simulink model "propeller"  (R2021a)
settings: Solver=VariableStepAuto  StartTime=0.0  StopTime=0.05  FixedStep=0.01  RelTol=1e-3
InitFcn:
  | prop_init_set
values from neighbouring files (symbols this model uses):
  Cp_total = [Cp_1000rpm; Cp_2000rpm; Cp_3000rpm; Cp_4000rpm; Cp_5000rpm]    [prop_init_set.m]
  Ct_total = [Ct_1000rpm; Ct_2000rpm; Ct_3000rpm; Ct_4000rpm; Ct_5000rpm]    [prop_init_set.m]
settings Model: SimulationMode=accelerator  Creator=76568  LastModifiedBy=76568

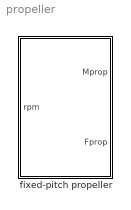
== system propeller ==
  fixed-pitch propeller : Subsystem  mask{air_speed=10, prop_diameter=0.473, T_static=16.1936, T_max=6.85, V_max=15, air_rho=1.225}

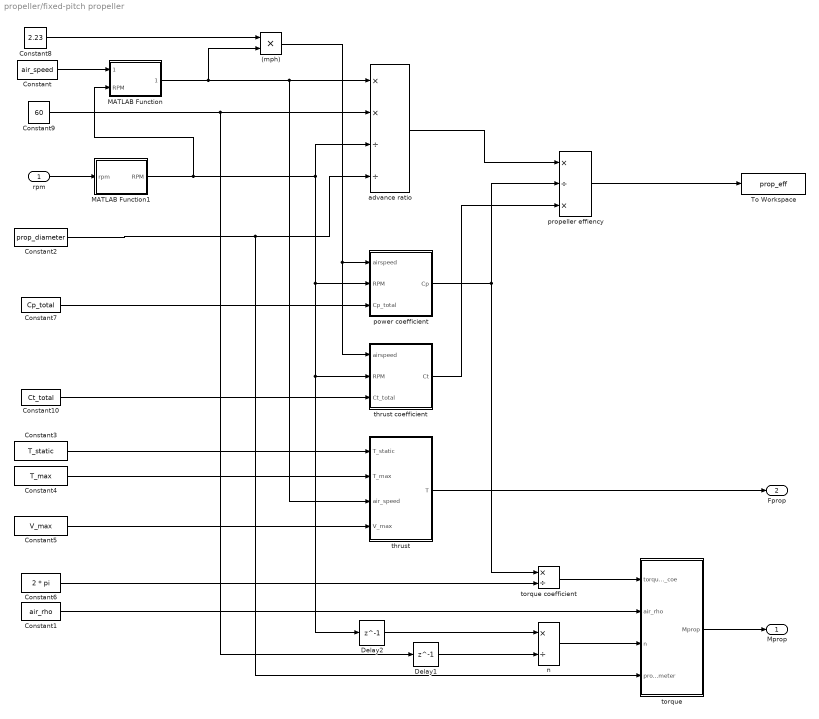
== system propeller/fixed-pitch propeller ==
  rpm : Inport
  (mph) : Product
  Constant : Constant  Value=air_speed
  Constant1 : Constant  Value=air_rho
  Constant10 : Constant  Value=Ct_total
  Constant2 : Constant  Value=prop_diameter
  Constant3 : Constant  Value=T_static
  Constant4 : Constant  Value=T_max
  Constant5 : Constant  Value=V_max
  Constant6 : Constant  Value=2 * pi
  Constant7 : Constant  Value=Cp_total
  Constant8 : Constant  Value=2.23
  Constant9 : Constant  Value=60
  Delay1 : Delay  DelayLength=1  InitialCondition=0  SampleTime=0.0001
  Delay2 : Delay  DelayLength=1  InitialCondition=0  SampleTime=0.0001
  MATLAB Function : MATLAB Function  TreatAsAtomicUnit=on
  MATLAB Function1 : MATLAB Function  TreatAsAtomicUnit=on
  To Workspace : ToWorkspace  VariableName=prop_eff  SaveFormat=Timeseries  SampleTime=-1
  advance ratio : Product  Inputs=**//
  n : Product  Inputs=*/
  power coefficient : MATLAB Function  TreatAsAtomicUnit=on
  propeller effiency : Product  Inputs=*/*
  thrust : MATLAB Function  TreatAsAtomicUnit=on
  thrust coefficient : MATLAB Function  TreatAsAtomicUnit=on
  torque : MATLAB Function  TreatAsAtomicUnit=on
  torque coefficient : Product  Inputs=*/
  Mprop : Outport
  Fprop : Outport  Port=2
  wires:
  thrust coefficient/1(Ct) -> propeller effiency/3
  MATLAB Function1/1(RPM) -> MATLAB Function/2(RPM), Delay2/1, thrust coefficient/2(RPM), power coefficient/2(RPM), advance ratio/3
  Constant2/1 -> advance ratio/4, torque/4(prop_diameter)
  advance ratio/1 -> propeller effiency/1
  torque coefficient/1 -> torque/1(torque_coe)
  Constant1/1 -> torque/2(air_rho)
  Constant10/1 -> thrust coefficient/3(Ct_total)
  MATLAB Function/1(airspeed) -> thrust/3(air_speed), advance ratio/1, (mph)/2
  Constant/1 -> MATLAB Function/1(air_speed)
  (mph)/1 -> thrust coefficient/1(airspeed), power coefficient/1(airspeed)
  Constant6/1 -> torque coefficient/2
  n/1 -> torque/3(n)
  Constant8/1 -> (mph)/1
  Constant7/1 -> power coefficient/3(Cp_total)
  Constant9/1 -> Delay1/1, advance ratio/2
  Constant3/1 -> thrust/1(T_static)
  rpm/1 -> MATLAB Function1/1(rpm)
  thrust/1(T) -> Fprop/1
  Constant5/1 -> thrust/4(V_max)
  propeller effiency/1 -> To Workspace/1
  Constant4/1 -> thrust/2(T_max)
  torque/1(Mprop) -> Mprop/1
  power coefficient/1(Cp) -> torque coefficient/1, propeller effiency/2
  Delay1/1 -> n/2
  Delay2/1 -> n/1

== matlab function propeller/fixed-pitch propeller/power coefficient ==
  data: airspeed input; Cp output; RPM input; Cp_total input
function Cp = fcn(airspeed, RPM, Cp_total)
Cp_temp = interp2(0 : 0.5 : 50, 1000 : 1000 : 5000, Cp_total, airspeed, RPM);
Cp_temp(isnan(Cp_temp)) = 0;
Cp = Cp_temp;

== matlab function propeller/fixed-pitch propeller/thrust ==
  data: T_static input; T output; T_max input; air_speed input; V_max input
function T = fcn(T_static, T_max, air_speed, V_max)
T = ((T_static - 2 * T_max) / V_max ^ 2) * air_speed ^ 2 + ((3 * T_max - 2 * T_static) / V_max) * air_speed + T_static;

== matlab function propeller/fixed-pitch propeller/thrust coefficient ==
  data: airspeed input; Ct output; RPM input; Ct_total input
function Ct = fcn(airspeed, RPM, Ct_total)
Ct_temp = interp2(0 : 0.5 : 50, 1000 : 1000 : 5000, Ct_total, airspeed, RPM);
Ct_temp(isnan(Ct_temp)) = 0;
Ct = Ct_temp;

== matlab function propeller/fixed-pitch propeller/torque ==
  data: torque_coe input; Mprop output; air_rho input; n input; prop_diameter input
function Mprop = fcn(torque_coe, air_rho, n, prop_diameter)
Mprop = torque_coe * air_rho * n ^ 2 * prop_diameter ^ 5;

== matlab function propeller/fixed-pitch propeller/MATLAB Function ==
  data: air_speed input; airspeed output; RPM input
function airspeed = fcn(air_speed, RPM)
if RPM <= 2000
    if air_speed > 8.94
       airspeed = 8.94;
    else
        airspeed = air_speed;
    end
end
if 2000 < RPM <= 3000
    if air_speed > 13.41
        airspeed = 13.41;
    else
        airspeed = air_speed;
    end
end
if 3000 < RPM <= 4000
    if air_speed > 17.88
        airspeed = 17.88;
    else
        airspeed = air_speed;
    end
end
if 4000 < RPM <= 5000
    if air_speed > 22.35
        airspeed = 22.35;
    else
        airspeed = air_speed;
    end
else
    airspeed = air_speed;
end
end

== matlab function propeller/fixed-pitch propeller/MATLAB Function1 ==
  data: rpm input; RPM output
function RPM = fcn(rpm)
if rpm < 1000
    rpm = 1000;
end
if rpm > 5000
    rpm = 5000;
end
RPM = rpm;
end
